simulink model "uz_mpc_6ph"  (R2024b)
settings: Solver=FixedStepDiscrete  StartTime=0.0  StopTime=0.003  RelTol=1e-3
values from neighbouring files (symbols this model uses):
  IB = sqrt(2)*IR    [uz_mpc_6ph_init.m]    (also in uz_mpc_6ph_state_machine_init.m)
  id_ref = 0.0    (= 0)    [uz_mpc_6ph_init.m]    (also in uz_mpc_6ph_state_machine_init.m)
  iq_ref = 15.0    (= 15)    [uz_mpc_6ph_init.m]    (also in uz_mpc_6ph_state_machine_init.m = 3)
  ix_ref = 0.0    (= 0)    [uz_mpc_6ph_init.m]    (also in uz_mpc_6ph_state_machine_init.m)
  iy_ref = 0.0    (= 0)    [uz_mpc_6ph_init.m]    (also in uz_mpc_6ph_state_machine_init.m)
  lambda_d = 1.0    (= 1)    [uz_mpc_6ph_init.m]    (also in uz_mpc_6ph_state_machine_init.m)
  lambda_q = 1.0    (= 1)    [uz_mpc_6ph_init.m]    (also in uz_mpc_6ph_state_machine_init.m)
  lambda_u = 0.0    (= 0)    [uz_mpc_6ph_init.m]    (also in uz_mpc_6ph_state_machine_init.m)
  lambda_x = 1.0    (= 1)    [uz_mpc_6ph_init.m]    (also in uz_mpc_6ph_state_machine_init.m)
  lambda_y = 1.0    (= 1)    [uz_mpc_6ph_init.m]    (also in uz_mpc_6ph_state_machine_init.m)
  Ld_over_LB = Ld/LB    [uz_mpc_6ph_init.m]    (also in uz_mpc_6ph_state_machine_init.m)
  Lq_over_LB = Lq/LB    [uz_mpc_6ph_init.m]    (also in uz_mpc_6ph_state_machine_init.m)
  n_rpm = 2200.0    (= 2200)    [uz_mpc_6ph_init.m]    (also in uz_mpc_6ph_state_machine_init.m = 1200)
  omegaB = nR*2*pi()/60*p    [uz_mpc_6ph_init.m]    (also in uz_mpc_6ph_state_machine_init.m)
  p = 5    [uz_mpc_6ph_init.m]    (also in uz_mpc_6ph_state_machine_init.m)
  psi_pm_over_psiB = psi_pm/psiB    [uz_mpc_6ph_init.m]    (also in uz_mpc_6ph_state_machine_init.m)
  Rs_over_ZB = Rs/ZB    [uz_mpc_6ph_init.m]    (also in uz_mpc_6ph_state_machine_init.m)
  t_ADC = 1/f_ADC    (= 1e-05)    [uz_mpc_6ph_init.m]    (also in uz_mpc_6ph_state_machine_init.m)
  t_clock = 1/f_clock    (= 1e-08)    [uz_mpc_6ph_init.m]    (also in uz_mpc_6ph_state_machine_init.m)
  Ts_times_ZB_over_Ld = Ts*ZB/Ld    [uz_mpc_6ph_init.m]    (also in uz_mpc_6ph_state_machine_init.m)
  Ts_times_ZB_over_Lq = Ts*ZB/Lq    [uz_mpc_6ph_init.m]    (also in uz_mpc_6ph_state_machine_init.m)
  Ts_times_ZB_over_Lx = Ts*ZB/Lx    [uz_mpc_6ph_init.m]    (also in uz_mpc_6ph_state_machine_init.m)
  Ts_times_ZB_over_Ly = Ts*ZB/Ly    [uz_mpc_6ph_init.m]    (also in uz_mpc_6ph_state_machine_init.m)
  v_dc = 565.0    (= 565)    [uz_mpc_6ph_init.m]    (also in uz_mpc_6ph_state_machine_init.m)
  VB = sqrt(2/3)*VR    [uz_mpc_6ph_init.m]    (also in uz_mpc_6ph_state_machine_init.m)
libraries: nesl_utility x32, fl_lib x29, simulink x23, ee_lib x12, hdlsllib x2, spsAlphaBetaZerotodq0Lib x1, batteryecm_lib x1
(part 1 of 4)
settings Model: DataTypeOverride=Off  Creator=micha  LastModifiedBy=hufnagelde
settings SolverCC: AlgebraicLoopSolver=TrustRegion
settings DataIOCC: LimitDataPoints=on  SaveOutput=off  SaveTime=off
settings OptimizationCC: BlockReduction=off  ConditionallyExecuteInputs=off  DefaultParameterBehavior=Inlined  LifeSpan=inf
settings DebuggingCC: AlgebraicLoopMsg=error  SingleTaskRateTransMsg=error  UnconnectedInputMsg=warning  UnconnectedOutputMsg=warning  UnconnectedLineMsg=warning  AllowSymbolicDim=off  StrictBusMsg=ErrorOnBusTreatedAsVector  SFUnexpectedBacktrackingDiag=warning  SFNoUnconditionalDefaultTransitionDiag=warning  SFExecutionAtInitializationDiag=none  ArithmeticOperatorsInVariantConditions=warning
settings HardwareCC: ProdBitPerPointer=32  ProdBitPerSizeT=32  ProdBitPerPtrDiffT=32  ProdLargestAtomicFloat=None  ProdIntDivRoundTo=Undefined  ProdEndianess=Unspecified  ProdWordSize=32  ProdHWDeviceType=ASIC/FPGA->ASIC/FPGA  ProdEqTarget=off
settings ModelReferenceCC: EnableRefExpFcnMdlSchedulingChecks=on
settings SFSimCC: SimUseLocalCustomCode=off  CustomCodeUndefinedFunction=UseInterfaceOnly
settings RTWCC: RTWUseLocalCustomCode=off  GPUComputeCapability=3.5  DLArmComputeVersion=19.05
settings CodeAppCC: StateflowObjectComments=on
settings GRTTargetCC: TargetLangStandard=C89/C90 (ANSI)
settings ConfigComp: CovScope=ReferencedModels  CovMetricSettings=dw  CovSaveCumulativeToWorkspaceVar=on  CovSaveSingleToWorkspaceVar=on  CovExternalEMLEnable=off  CovSFcnEnable=off

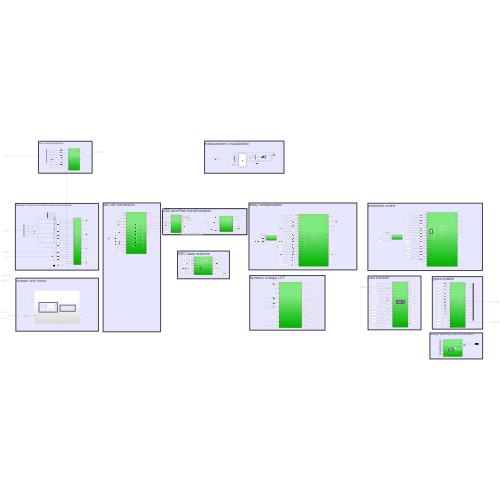
[thumbnail: Simulink's stored preview of the top-level diagram]
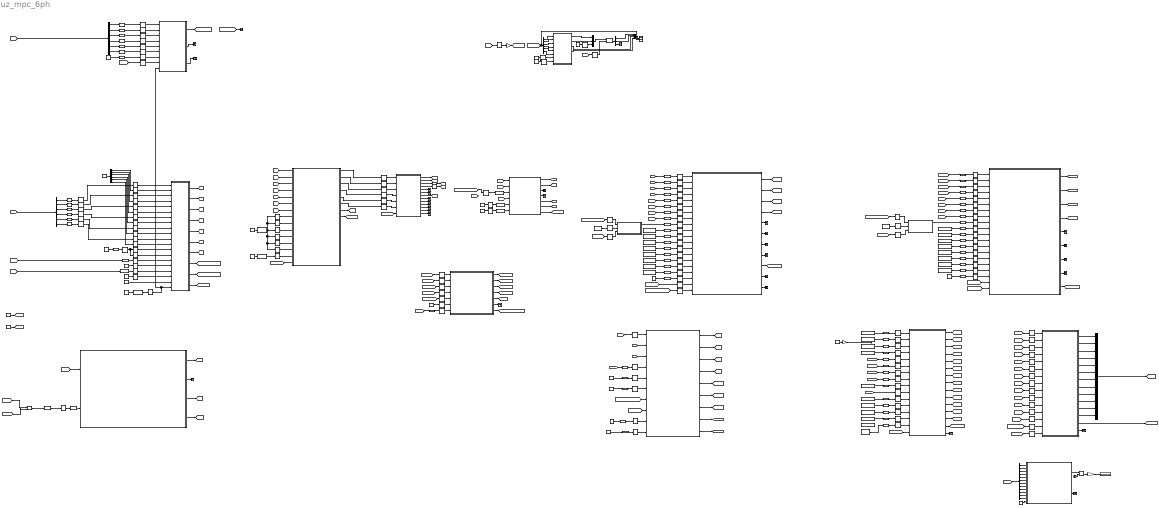
== system uz_mpc_6ph ==
  note: measurement visualization
  note: sfix27_En24 = +-4 p.u.
  note: current limit in A
  note: inverter and motor
  note: debug ip for input of constant measurement values
  note: VSD and Park transformation
  note: MPC state machine
  note: per unit conversion
  note: average switching frequency calculation
  note: gates enable
  note: cost function
  note: prediction model
  note: dynamic voltage LUT
  note: delay compensation
  note: 1=real 0=debug
  note: 5 steps delay for xy currents, since dq transformation of alpha beta currents takes 5 clock steps. This way, the delay of dq is compensated. For implementation not relevant!
  note: 0=AXI 1=PL
  note: 0=AXI 1=PL
  note: over current protection
  6ph_PMSM_30deg_VSD1 : MATLAB Function  TreatAsAtomicUnit=on
  AND : Logic  IconShape=distinctive  AllPortsSameDT=off  OutDataTypeStr=boolean
  Alpha-Beta-Zero to dq1 : spsAlphaBetaZerotodq0Lib/Alpha-Beta-Zero to dq0  Alignment=Aligned with phase A axis
  Clock : Clock
  Constant : Constant  Value=64  OutDataTypeStr=uint32  SampleTime=-1
  Constant1 : Constant  Value=p
  Constant10 : Constant  Value=psi_pm_over_psiB
  Constant11 : Constant  Value=1.2
  Constant12 : Constant  Value=0
  Constant13 : Constant  Value=p
  Constant14 : Constant  Value=psi_pm_over_psiB
  Constant15 : Constant  Value=Rs_over_ZB
  Constant16 : Constant  Value=12
  Constant17 : Constant  Value=Ts_times_ZB_over_Ld
  Constant18 : Constant  Value=Ts_times_ZB_over_Lq
  Constant19 : Constant  Value=Ts_times_ZB_over_Lx
  Constant{2,25,51,62} (4 alike) : Constant
  Constant20 : Constant  Value=Ts_times_ZB_over_Ly
  Constant21 : Constant  Value=Ld_over_LB
  Constant22 : Constant  Value=Lq_over_LB
  Constant23 : Constant  Value=39
  Constant24 : Constant  Value=1/3
  Constant26 : Constant  Value=v_dc
  Constant27 : Constant  Value=iq_ref/IB
  Constant28 : Constant  Value=ix_ref/IB
  Constant29 : Constant  Value=iy_ref/IB
  Constant3 : Constant  Value=Rs_over_ZB
  Constant30 : Constant  Value=0  SampleTime=-1
  Constant31 : Constant  Value=lambda_d
  Constant32 : Constant  Value=lambda_q
  Constant33 : Constant  Value=lambda_x
  Constant34 : Constant  Value=lambda_y
  Constant35 : Constant  Value=lambda_u
  Constant36 : Constant  OutDataTypeStr=boolean  SampleTime=-1
  Constant37 : Constant  OutDataTypeStr=boolean  SampleTime=-1
  Constant4 : Constant  Value=Ts_times_ZB_over_Ld
  Constant42 : Constant  Value=id_ref/IB
  Constant44 : Constant  Value=0  SampleTime=-1
  Constant5 : Constant  Value=Ts_times_ZB_over_Lq
  Constant52 : Constant  Value=0
  Constant53 : Constant  Value=1/omegaB  OutDataTypeStr=fixdt(0,18,18)
  Constant54 : Constant  Value=1/omegaB  OutDataTypeStr=fixdt(0,18,18)
  Constant55 : Constant  Value=0  OutDataTypeStr=fixdt(1,24,11)  SampleTime=-1
  Constant56 : Constant  Value=1/IB
  Constant57 : Constant  Value=1/VB
  Constant58 : Constant  Value=63
  Constant59 : Constant  OutDataTypeStr=boolean  SampleTime=-1
  Constant6 : Constant  Value=Ts_times_ZB_over_Lx
  Constant60 : Constant  Value=[1 2 3 4 5 6]  OutDataTypeStr=fixdt(1,27,15)  SampleTime=-1
  Constant61 : Constant  Value=0  OutDataTypeStr=fixdt(1,27,20)  SampleTime=-1
  Constant63 : Constant  Value=0.15
  Constant7 : Constant  Value=Ts_times_ZB_over_Ly
  Constant8 : Constant  Value=Ld_over_LB
  Constant9 : Constant  Value=Lq_over_LB
  Data Type Conversion{,3,55..58} (6 alike) : DataTypeConversion  OutDataTypeStr=fixdt_type_xy_currents  SaturateOnIntegerOverflow=off  RndMeth=Floor
  Data Type Conversion1 : DataTypeConversion  OutDataTypeStr=boolean  SaturateOnIntegerOverflow=off  RndMeth=Floor
  Data Type Conversion{2,6,10..11,13,65..66} (7 alike) : DataTypeConversion  OutDataTypeStr=fixdt_type_polepairs  SaturateOnIntegerOverflow=off  RndMeth=Floor
  Data Type Conversion{12,14..28} (16 alike) : DataTypeConversion  OutDataTypeStr=fixdt_type_constants  SaturateOnIntegerOverflow=off  RndMeth=Floor
  Data Type Conversion29 : DataTypeConversion  OutDataTypeStr=fixdt_type_speed  SaturateOnIntegerOverflow=off  RndMeth=Floor
  Data Type Conversion30 : DataTypeConversion  OutDataTypeStr=fixdt_type_speed  SaturateOnIntegerOverflow=off  RndMeth=Floor
  Data Type Conversion{4..5,31,43..45,50..53} (10 alike) : DataTypeConversion  OutDataTypeStr=fixdt_type_dq_currents  SaturateOnIntegerOverflow=off  RndMeth=Floor
  Data Type Conversion32 : DataTypeConversion  OutDataTypeStr=fixdt(0,18,18)  SaturateOnIntegerOverflow=off  RndMeth=Floor
  Data Type Conversion33 : DataTypeConversion  OutDataTypeStr=fixdt(0,18,18)  SaturateOnIntegerOverflow=off  RndMeth=Floor
  Data Type Conversion{34..36,38,40,67..68,71..77} (14 alike) : DataTypeConversion  OutDataTypeStr=fixdt(1,27,15)  SaturateOnIntegerOverflow=off  RndMeth=Floor
  Data Type Conversion37 : DataTypeConversion  OutDataTypeStr=fixdt(1,27,20)  SaturateOnIntegerOverflow=off  RndMeth=Floor
  Data Type Conversion39 : DataTypeConversion  OutDataTypeStr=fixdt(1,18,14)  SaturateOnIntegerOverflow=off  RndMeth=Floor
  Data Type Conversion{7..8,41..42,46..49} (8 alike) : DataTypeConversion  OutDataTypeStr=fixdt_type_dqxy_voltages  SaturateOnIntegerOverflow=off  RndMeth=Floor
  Data Type Conversion54 : DataTypeConversion  OutDataTypeStr=fixdt_type_max_current  SaturateOnIntegerOverflow=off  RndMeth=Floor
  Data Type Conversion59 : DataTypeConversion  OutDataTypeStr=fixdt(1,18,14)  SaturateOnIntegerOverflow=off  RndMeth=Floor
  Data Type Conversion{60..64} (5 alike) : DataTypeConversion  OutDataTypeStr=fixdt_type_lambda  SaturateOnIntegerOverflow=off  RndMeth=Floor
  Data Type Conversion69 : DataTypeConversion  OutDataTypeStr=fixdt(1,24,11)  SaturateOnIntegerOverflow=off  RndMeth=Floor
  Data Type Conversion70 : DataTypeConversion  OutDataTypeStr=fixdt(1,18,15)  SaturateOnIntegerOverflow=off  RndMeth=Floor
  Data Type Conversion78 : DataTypeConversion  OutDataTypeStr=double  SaturateOnIntegerOverflow=off  RndMeth=Floor
  Data Type Conversion79 : DataTypeConversion  OutDataTypeStr=boolean  SaturateOnIntegerOverflow=off  RndMeth=Floor
  Data Type Conversion9 : DataTypeConversion  OutDataTypeStr=fixdt(1,27,20)  SaturateOnIntegerOverflow=off  RndMeth=Floor
  Delay3 : Delay  DelayLength=5
  Delay4 : Delay  DelayLength=5
  Demux{,1,5..6} (4 alike) : Demux  Outputs=6
  Demux2 : Demux  Outputs=12
  Demux4 : Demux  Outputs=3
  Display : Display
  Divide : Product  Inputs=*/
  Gain : Gain  Gain=1/IB
  Gain1 : Gain  Gain=1/IB
  Gain19 : Gain  Gain=1/(12*2)
  Mux : Mux
  Mux2 : Mux  Inputs=12
  Mux5 : Mux  Inputs=3
  Pulse Generator2 : DiscretePulseGenerator  PulseType=Time based  Period=t_ADC  PulseWidth=5
  Rate Transition{,5,8,131..132} (5 alike) : RateTransition  OutPortSampleTime=t_ADC
  Rate Transition{1..4,6..7,9..10,12..54,56..67,69..74,77..128,130,133..141} (131 alike) : RateTransition  OutPortSampleTime=t_clock
  Rate Transition{11,55,68,75..76,129} (6 alike) : RateTransition  InitialCondition=1  OutPortSampleTime=t_clock
  Scope : Scope  NumInputPorts=2
  Terminator{,1..28} (29 alike) : Terminator
  Transport Delay : TransportDelay  DelayTime=0.0015  InitialOutput=1
  cost_opt : Subsystem  TreatAsAtomicUnit=on
  counter_f_sw_6ph : Subsystem
  ctrl_state_machine : Subsystem  TreatAsAtomicUnit=on
  delay_comp : Subsystem  TreatAsAtomicUnit=on
  inverter_machine : Subsystem
  mpc_enable : Subsystem  TreatAsAtomicUnit=on
  prediction : Subsystem  TreatAsAtomicUnit=on
  pu_omega_m : Subsystem  TreatAsAtomicUnit=on
  pu_omega_m1 : Subsystem
  pu_voltages_vsd : Subsystem  TreatAsAtomicUnit=on
  uz_current_limit : Subsystem  TreatAsAtomicUnit=on
  uz_debug_switch_measurements : Subsystem  TreatAsAtomicUnit=on
  uz_park_transformation : Subsystem  TreatAsAtomicUnit=on
  uz_pu_conversion : Subsystem  TreatAsAtomicUnit=on
  uz_vsd_6ph_30deg : Subsystem  TreatAsAtomicUnit=on
  wires:
  [optimization_done] -> Rate Transition4/1
  [prediction_done] -> Rate Transition3/1
  [delay_comp_done] -> Rate Transition2/1
  [voltages_done] -> Rate Transition1/1
  Rate Transition58/1 -> ctrl_state_machine/1(trigger_start_state_machine)  "park_done"
  Rate Transition1/1 -> ctrl_state_machine/2(trigger_voltages_done)  "volts_done"
  Rate Transition2/1 -> ctrl_state_machine/3(trigger_delay_comp_done)  "delay_done"
  Rate Transition3/1 -> ctrl_state_machine/4(trigger_prediction_done)  "pred_done"
  Rate Transition4/1 -> ctrl_state_machine/5(trigger_optimization_done)  "opt_done"
  Rate Transition9/1 -> ctrl_state_machine/6(AXI_no_of_iterations)  "opt_done"
  Constant/1 -> Rate Transition9/1
  uz_park_transformation/7(park_done) -> [trigger_park_done]  "calc_done"
  Rate Transition36/1 -> uz_vsd_6ph_30deg/5(b2)
  Rate Transition38/1 -> Data Type Conversion9/1
  Data Type Conversion39/1 -> uz_park_transformation/5(factor_angle_el_AXI)
  uz_park_transformation/3(y1_AXI) -> Terminator8/1
  uz_vsd_6ph_30deg/8(alpha_AXI) -> Terminator2/1
  Data Type Conversion9/1 -> uz_park_transformation/3(angle_el)
  uz_park_transformation/2(y2) -> [iq_pu]  "iq_pu"
  Data Type Conversion59/1 -> uz_park_transformation/6(offset_angle_el_AXI)
  uz_vsd_6ph_30deg/3(x1) -> Delay3/1
  Demux/4 -> Data Type Conversion38/1
  Rate Transition61/1 -> Data Type Conversion59/1
  Rate Transition40/1 -> Data Type Conversion39/1
  uz_vsd_6ph_30deg/4(y1) -> Delay4/1
  Constant12/1 -> Rate Transition61/1
  uz_vsd_6ph_30deg/5(z1) -> Terminator/1
  uz_vsd_6ph_30deg/6(z2) -> Terminator1/1
  uz_vsd_6ph_30deg/13(z2_AXI) -> Terminator7/1
  Demux/2 -> Data Type Conversion35/1
  Rate Transition33/1 -> uz_vsd_6ph_30deg/3(c1)
  uz_park_transformation/1(y1) -> [id_pu]  "id_pu"
  uz_vsd_6ph_30deg/10(x_AXI) -> Terminator4/1
  inverter_machine/4(omega_m) -> [omega_m]
  inverter_machine/3(theta_el) -> [theta_el]
  inverter_machine/2(i_dc) -> Terminator25/1
  uz_vsd_6ph_30deg/9(beta_AXI) -> Terminator3/1
  uz_park_transformation/5(sin) -> [sin]
  inverter_machine/1(i_ph) -> [i_ph]
  uz_vsd_6ph_30deg/12(z1_AXI) -> Terminator6/1
  [i_ph] -> Demux/1
  Rate Transition35/1 -> uz_vsd_6ph_30deg/1(a1)
  Constant25/1 -> Rate Transition40/1
  Demux/6 -> Data Type Conversion67/1
  Demux/5 -> Data Type Conversion40/1
  Demux/3 -> Data Type Conversion36/1
  Rate Transition32/1 -> uz_vsd_6ph_30deg/2(b1)
  Demux/1 -> Data Type Conversion34/1
  uz_pu_conversion/8(pu_conv_done) -> [pu_conv_valid]
  Data Type Conversion1/1 -> Rate Transition10/1
  uz_vsd_6ph_30deg/11(y_AXI) -> Terminator5/1
  Rate Transition34/1 -> uz_vsd_6ph_30deg/4(a2)
  Pulse Generator2/1 -> Data Type Conversion1/1
  uz_park_transformation/6(cos) -> [cos]
  [theta_el_from_debug_switch] -> Rate Transition38/1
  uz_park_transformation/4(y2_AXI) -> Terminator9/1
  Constant13/1 -> Data Type Conversion11/1
  Constant14/1 -> Data Type Conversion27/1
  Data Type Conversion16/1 -> Rate Transition14/1
  Data Type Conversion12/1 -> Rate Transition13/1
  Data Type Conversion65/1 -> Rate Transition55/1
  Rate Transition15/1 -> delay_comp/18(polepairs_AXI)
  pu_voltages_vsd/9(voltages_done) -> [voltages_done]  "calc_done"
  pu_voltages_vsd/1(pu_vd) -> [vd_pu]
  [v_dc_pu] -> Rate Transition46/1
  Constant22/1 -> Data Type Conversion19/1
  Rate Transition74/1 -> delay_comp/6(vq_pu)
  Rate Transition47/1 -> delay_comp/7(vx_pu)
  Data Type Conversion41/1 -> Rate Transition47/1
  Rate Transition51/1 -> prediction/7(vx_pu)
  Data Type Conversion14/1 -> Rate Transition20/1
  Rate Transition19/1 -> prediction/17(psi_pm_over_psiB_AXI)
  Constant15/1 -> Data Type Conversion12/1
  Constant21/1 -> Data Type Conversion18/1
  Constant18/1 -> Data Type Conversion15/1
  pu_omega_m1/1(out1) -> Data Type Conversion30/1
  Data Type Conversion21/1 -> Rate Transition39/1
  Constant8/1 -> Data Type Conversion25/1
  Rate Transition75/1 -> pu_voltages_vsd/4(index)
  [vq_pu] -> Data Type Conversion8/1
  delay_comp/9(delay_comp_done) -> [delay_comp_done]
  Data Type Conversion18/1 -> Rate Transition17/1
  pu_voltages_vsd/2(pu_vq) -> [vq_pu]
  Data Type Conversion45/1 -> Rate Transition50/1
  Rate Transition24/1 -> prediction/4(iy_delay_pu)
  Rate Transition26/1 -> delay_comp/13(Ts_times_ZB_over_Lx_AXI)
  Constant2/1 -> Data Type Conversion2/1
  [cos] -> pu_voltages_vsd/3(cos_angle)
  Rate Transition46/1 -> pu_voltages_vsd/1(v_DC_pu)
  Constant30/1 -> counter_f_sw_6ph/13(bResetAXI)
  Data Type Conversion31/1 -> Rate Transition49/1
  [iq_delay_pu] -> Data Type Conversion45/1
  Data Type Conversion15/1 -> Rate Transition21/1
  counter_f_sw_6ph/1(switchNumb_AXI) -> Divide/1
  Rate Transition48/1 -> delay_comp/8(vy_pu)
  Rate Transition21/1 -> prediction/12(Ts_times_ZB_over_Lq_AXI)
  Constant17/1 -> Data Type Conversion14/1
  pu_voltages_vsd/5(pu_vd_AXI) -> [vd_pu_AXI]
  Data Type Conversion47/1 -> Rate Transition52/1
  Rate Transition50/1 -> prediction/2(iq_delay_pu)
  cost_opt/15(costs) -> Terminator10/1
  Rate Transition67/1 -> delay_comp/5(vd_pu)
  Demux2/11 -> counter_f_sw_6ph/11(ss_in_10)
  [opt_gates] -> Demux2/1
  Data Type Conversion30/1 -> Rate Transition23/1
  Demux2/2 -> counter_f_sw_6ph/2(ss_in_1)
  Rate Transition44/1 -> delay_comp/3(ix_pu)
  Constant9/1 -> Data Type Conversion26/1
  Clock/1 -> Divide/2
  Data Type Conversion42/1 -> Rate Transition48/1
  Demux2/3 -> counter_f_sw_6ph/3(ss_in_2)
  Demux2/10 -> counter_f_sw_6ph/10(ss_in_9)
  Data Type Conversion58/1 -> Rate Transition66/1
  Data Type Conversion4/1 -> Rate Transition41/1
  [index] -> Data Type Conversion6/1
  Demux2/1 -> counter_f_sw_6ph/1(ss_in_0)
  Rate Transition18/1 -> prediction/16(Lq_over_LB_AXI)
  Rate Transition68/1 -> cost_opt/10(index)
  Rate Transition52/1 -> prediction/8(vy_pu)
  pu_voltages_vsd/3(pu_vx) -> [vx_pu]
  Data Type Conversion57/1 -> Rate Transition65/1
  Rate Transition11/1 -> pu_voltages_vsd/5(index_select_AXI)
  Demux2/6 -> counter_f_sw_6ph/6(ss_in_5)
  Constant20/1 -> Data Type Conversion17/1
  Gain19/1 -> Display/1
  Data Type Conversion28/1 -> Rate Transition31/1
  Demux2/12 -> counter_f_sw_6ph/12(ss_in_11)
  Rate Transition69/1 -> cost_opt/11(lambda_d_AXI)
  Rate Transition54/1 -> prediction/6(vq_pu)
  [sin] -> pu_voltages_vsd/2(sin_angle)
  Demux2/7 -> counter_f_sw_6ph/7(ss_in_6)
  prediction/4(iy_pred_pu) -> [iy_pred_pu]
  Demux2/8 -> counter_f_sw_6ph/8(ss_in_7)
  pu_voltages_vsd/7(pu_vx_AXI) -> [vx_pu_AXI]
  Rate Transition70/1 -> cost_opt/12(lambda_q_AXI)
  pu_voltages_vsd/6(pu_vq_AXI) -> [vq_pu_AXI]
  [index] -> Rate Transition68/1
  Data Type Conversion27/1 -> Rate Transition19/1
  pu_voltages_vsd/8(pu_vy_AXI) -> [vy_pu_AXI]
  [vd_pu] -> Data Type Conversion7/1
  Data Type Conversion43/1 -> Rate Transition24/1
  Constant32/1 -> Data Type Conversion61/1
  Constant11/1 -> Data Type Conversion54/1
  Data Type Conversion19/1 -> Rate Transition18/1
  Data Type Conversion10/1 -> Rate Transition76/1
  Constant19/1 -> Data Type Conversion16/1
  Data Type Conversion48/1 -> Rate Transition53/1
  Rate Transition12/1 -> prediction/18(polepairs_AXI)
  Rate Transition20/1 -> prediction/11(Ts_times_ZB_over_Ld_AXI)
  Rate Transition29/1 -> delay_comp/15(Ld_over_LB_AXI)
  Rate Transition17/1 -> prediction/15(Ld_over_LB_AXI)
  pu_voltages_vsd/4(pu_vy) -> [vy_pu]
  Data Type Conversion13/1 -> Rate Transition15/1
  [opt_index] -> Data Type Conversion10/1
  Rate Transition22/1 -> delay_comp/4(iy_pu)
  Rate Transition43/1 -> delay_comp/9(omega_m_pu)
  Data Type Conversion11/1 -> Rate Transition12/1
  Constant10/1 -> Data Type Conversion28/1
  Data Type Conversion51/1 -> Rate Transition56/1
  [iy_pu] -> Data Type Conversion3/1
  [vd_pu] -> Data Type Conversion48/1
  Data Type Conversion17/1 -> Rate Transition16/1
  Data Type Conversion46/1 -> Rate Transition51/1
  Data Type Conversion3/1 -> Rate Transition22/1
  Constant1/1 -> Data Type Conversion13/1
  prediction/9(prediction_done) -> [prediction_done]
  Constant33/1 -> Data Type Conversion62/1
  Rate Transition53/1 -> prediction/5(vd_pu)
  cost_opt/1(opt_index) -> [opt_index]  "result"
  Rate Transition13/1 -> prediction/10(Rs_over_ZB_AXI)
  [iq_pu] -> Data Type Conversion5/1
  Constant34/1 -> Data Type Conversion63/1
  Data Type Conversion20/1 -> Rate Transition25/1
  Rate Transition60/1 -> cost_opt/6(iq_pred_pu)
  cost_opt/14(optimization_done) -> [optimization_done]  "optimization done"
  Data Type Conversion56/1 -> Rate Transition64/1
  Constant44/1 -> Data Type Conversion64/1
  Constant4/1 -> Data Type Conversion21/1
  Rate Transition73/1 -> cost_opt/15(lambda_u_AXI)
  Data Type Conversion64/1 -> Rate Transition73/1
  Demux2/4 -> counter_f_sw_6ph/4(ss_in_3)
  Data Type Conversion61/1 -> Rate Transition70/1
  Data Type Conversion22/1 -> Rate Transition42/1
  Rate Transition76/1 -> ctrl_state_machine/7(last_opt_index)
  Data Type Conversion60/1 -> Rate Transition69/1
  Constant42/1 -> Data Type Conversion57/1
  Rate Transition71/1 -> cost_opt/13(lambda_x_AXI)
  Rate Transition72/1 -> cost_opt/14(lambda_y_AXI)
  Rate Transition63/1 -> cost_opt/3(ix_ref_pu_AXI)
  Constant5/1 -> Data Type Conversion22/1
  Rate Transition64/1 -> cost_opt/4(iy_ref_pu_AXI)
  Rate Transition65/1 -> cost_opt/1(id_ref_pu_AXI)
  Rate Transition16/1 -> prediction/14(Ts_times_ZB_over_Ly_AXI)
  [vy_pu] -> Data Type Conversion42/1
  Divide/1 -> Gain19/1
  [vx_pu] -> Data Type Conversion41/1
  Rate Transition57/1 -> cost_opt/5(id_pred_pu)
  Rate Transition23/1 -> prediction/9(omega_m_pu)
  Gain1/1 -> ?
  Data Type Conversion6/1 -> Rate Transition75/1
  [iq_pred_pu] -> Data Type Conversion53/1
  Rate Transition28/1 -> prediction/1(id_delay_pu)
  Rate Transition55/1 -> pu_voltages_vsd/6(index_AXI)
  Data Type Conversion63/1 -> Rate Transition72/1
  Constant6/1 -> Data Type Conversion23/1
  Rate Transition59/1 -> cost_opt/7(ix_pred_pu)
  Data Type Conversion55/1 -> Rate Transition63/1
  Data Type Conversion44/1 -> Rate Transition28/1
  [ix_pred_pu] -> Data Type Conversion50/1
  [id_pred_pu] -> Data Type Conversion52/1
  Rate Transition31/1 -> delay_comp/17(psi_pm_over_psiB_AXI)
  Data Type Conversion52/1 -> Rate Transition57/1
  Data Type Conversion49/1 -> Rate Transition54/1
  Data Type Conversion8/1 -> Rate Transition74/1
  [id_delay_pu] -> Data Type Conversion44/1
  [id_pu] -> Data Type Conversion4/1
  Data Type Conversion62/1 -> Rate Transition71/1
  [iy_delay_pu] -> Data Type Conversion43/1
  Rate Transition66/1 -> cost_opt/2(iq_ref_pu_AXI)
  [ix_delay_pu] -> Data Type Conversion31/1
  Data Type Conversion53/1 -> Rate Transition60/1
  counter_f_sw_6ph/2(switchNumb) -> Terminator24/1
  [ix_pu] -> Data Type Conversion/1
  Data Type Conversion54/1 -> Rate Transition62/1
  prediction/3(ix_pred_pu) -> [ix_pred_pu]
  Data Type Conversion24/1 -> Rate Transition27/1
  [vx_pu] -> Data Type Conversion46/1
  [iy_pred_pu] -> Data Type Conversion51/1
  [vq_pu] -> Data Type Conversion49/1
  Data Type Conversion2/1 -> Rate Transition11/1
  prediction/1(id_pred_pu) -> [id_pred_pu]
  Constant28/1 -> Data Type Conversion55/1
  Data Type Conversion/1 -> Rate Transition44/1
  Rate Transition25/1 -> delay_comp/10(Rs_over_ZB_AXI)
  Demux2/5 -> counter_f_sw_6ph/5(ss_in_4)
  [vy_pu] -> Data Type Conversion47/1
  Data Type Conversion5/1 -> Rate Transition45/1
  Data Type Conversion23/1 -> Rate Transition26/1
  Constant3/1 -> Data Type Conversion20/1
  Data Type Conversion26/1 -> Rate Transition30/1
  Rate Transition27/1 -> delay_comp/14(Ts_times_ZB_over_Ly_AXI)
  Rate Transition42/1 -> delay_comp/12(Ts_times_ZB_over_Lq_AXI)
  Rate Transition14/1 -> prediction/13(Ts_times_ZB_over_Lx_AXI)
  Constant31/1 -> Data Type Conversion60/1
  Rate Transition30/1 -> delay_comp/16(Lq_over_LB_AXI)
  Data Type Conversion25/1 -> Rate Transition29/1
  Rate Transition56/1 -> cost_opt/8(iy_pred_pu)
  Demux2/9 -> counter_f_sw_6ph/9(ss_in_8)
  Data Type Conversion50/1 -> Rate Transition59/1
  Data Type Conversion7/1 -> Rate Transition67/1
  Constant7/1 -> Data Type Conversion24/1
  pu_omega_m/1(out1) -> Data Type Conversion29/1
  Rate Transition45/1 -> delay_comp/2(iq_pu)
  Rate Transition49/1 -> prediction/3(ix_delay_pu)
  Data Type Conversion29/1 -> Rate Transition43/1
  Rate Transition62/1 -> cost_opt/9(max_current_pu_AXI)
  Rate Transition39/1 -> delay_comp/11(Ts_times_ZB_over_Ld_AXI)
  Constant29/1 -> Data Type Conversion56/1
  [trigger_park_done] -> Rate Transition58/1
  [delay_comp_done] -> prediction/20(trigger_delay_comp_done)
  [trigger_park_done_statemachine] -> pu_voltages_vsd/7(trigger_park_done)
  ctrl_state_machine/5(index) -> [index]
  Rate Transition37/1 -> uz_vsd_6ph_30deg/6(c2)
  Rate Transition41/1 -> delay_comp/1(id_pu)  "id_measured"
  [opt_gates] -> inverter_machine/1(In1)
  delay_comp/1(id_delay_pu) -> [id_delay_pu]  "id_delay"
  delay_comp/2(iq_delay_pu) -> [iq_delay_pu]
  delay_comp/4(iy_delay_pu) -> [iy_delay_pu]
  delay_comp/3(ix_delay_pu) -> [ix_delay_pu]
  ctrl_state_machine/7(trigger_park_done_statemachine) -> [trigger_park_done_statemachine]
  [trigger_park_done_statemachine] -> Rate Transition6/1
  Rate Transition6/1 -> delay_comp/20(trigger_park_done)
  Rate Transition7/1 -> delay_comp/19(trigger_delay_comp)
  Delay3/1 -> [ix_pu]
  Delay4/1 -> [iy_pu]
  Demux5/4 -> 6ph_PMSM_30deg_VSD1/4(u4)
  Demux5/5 -> 6ph_PMSM_30deg_VSD1/5(u5)
  Demux5/2 -> 6ph_PMSM_30deg_VSD1/2(u2)
  Demux5/3 -> 6ph_PMSM_30deg_VSD1/3(u3)
  Constant51/1 -> Rate Transition8/1
  [pu_phase_currents] -> Scope/2, Demux5/1
  Constant24/1 -> Rate Transition5/1
  Demux5/1 -> 6ph_PMSM_30deg_VSD1/1(u1)
  Demux5/6 -> 6ph_PMSM_30deg_VSD1/6(u6)
  [i_ph] -> Rate Transition/1
  Gain/1 -> [pu_phase_currents]
  Constant52/1 -> Rate Transition131/1
  [theta_el] -> Rate Transition132/1
  6ph_PMSM_30deg_VSD1/1(y1) -> Mux5/1  "alpha"
  Mux5/1 -> Alpha-Beta-Zero to dq1/1
  Alpha-Beta-Zero to dq1/1 -> Demux4/1
  6ph_PMSM_30deg_VSD1/2(y2) -> Mux5/2  "beta"
  Demux4/3 -> Terminator11/1
  [omega_m_from_debug_switch] -> Rate Transition79/1
  [pu_conv_valid] -> Rate Transition77/1
  Constant53/1 -> Rate Transition78/1
  Rate Transition77/1 -> pu_omega_m/3(adc_valid_trigger)
  Rate Transition78/1 -> pu_omega_m/2(AXI_pu_conv_in)
  Rate Transition79/1 -> pu_omega_m/1(in1)
  Rate Transition80/1 -> pu_omega_m1/3(adc_valid_trigger)
  Rate Transition82/1 -> pu_omega_m1/1(in1)
  [pu_conv_valid] -> Rate Transition80/1
  Constant54/1 -> Rate Transition81/1
  Rate Transition81/1 -> pu_omega_m1/2(AXI_pu_conv_in)
  [omega_m_from_debug_switch] -> Rate Transition82/1
  mpc_enable/10(out_G9) -> Mux2/10
  Mux2/1 -> [opt_gates]
  mpc_enable/1(out_G0) -> Mux2/1
  mpc_enable/2(out_G1) -> Mux2/2
  mpc_enable/5(out_G4) -> Mux2/5
  mpc_enable/3(out_G2) -> Mux2/3
  mpc_enable/6(out_G5) -> Mux2/6
  mpc_enable/12(out_G11) -> Mux2/12
  mpc_enable/7(out_G6) -> Mux2/7
  mpc_enable/11(out_G10) -> Mux2/11
  mpc_enable/9(out_G8) -> Mux2/9
  mpc_enable/4(out_G3) -> Mux2/4
  mpc_enable/8(out_G7) -> Mux2/8
  [pu_conv_valid] -> Rate Transition86/1
  [MPC_enb] -> Rate Transition85/1
  Rate Transition83/1 -> mpc_enable/11(G10)
  Rate Transition84/1 -> mpc_enable/12(G11)
  Rate Transition85/1 -> mpc_enable/13(AXI_mpc_enb)
  Rate Transition86/1 -> mpc_enable/15(adc_valid_trigger)
  Rate Transition87/1 -> mpc_enable/9(G8)
  Rate Transition88/1 -> mpc_enable/10(G9)
  Rate Transition89/1 -> mpc_enable/7(G6)
  Rate Transition90/1 -> mpc_enable/8(G7)
  Rate Transition91/1 -> mpc_enable/5(G4)
  Rate Transition92/1 -> mpc_enable/6(G5)
  Rate Transition94/1 -> mpc_enable/4(G3)
  Rate Transition93/1 -> mpc_enable/3(G2)
  Rate Transition95/1 -> mpc_enable/1(G0)
  Rate Transition96/1 -> mpc_enable/2(G1)
  Constant26/1 -> Data Type Conversion68/1
  Rate Transition106/1 -> uz_pu_conversion/8(AXI_pu_conv_in0)
  Rate Transition105/1 -> uz_pu_conversion/9(AXI_pu_conv_in1)
  Rate Transition104/1 -> uz_pu_conversion/10(AXI_pu_conv_in2)
  Rate Transition110/1 -> uz_pu_conversion/11(AXI_pu_conv_in3)
  Rate Transition109/1 -> uz_pu_conversion/12(AXI_pu_conv_in4)
  Rate Transition108/1 -> uz_pu_conversion/13(AXI_pu_conv_in5)
  Rate Transition107/1 -> uz_pu_conversion/14(AXI_pu_conv_in6)
  Constant56/1 -> Data Type Conversion33/1
  Constant57/1 -> Data Type Conversion32/1
  Data Type Conversion32/1 -> Rate Transition107/1
  Data Type Conversion33/1 -> Rate Transition106/1, Rate Transition105/1, Rate Transition104/1, Rate Transition110/1, Rate Transition109/1, Rate Transition108/1
  Data Type Conversion34/1 -> Rate Transition102/1
  Data Type Conversion35/1 -> Rate Transition101/1
  Data Type Conversion36/1 -> Rate Transition100/1
  Data Type Conversion38/1 -> Rate Transition99/1
  Data Type Conversion40/1 -> Rate Transition98/1
  Data Type Conversion67/1 -> Rate Transition97/1
  Data Type Conversion68/1 -> Rate Transition103/1
  uz_pu_conversion/7(out6) -> [v_dc_pu]
  Constant58/1 -> Data Type Conversion65/1
  uz_pu_conversion/1(out0) -> Rate Transition35/1
  uz_pu_conversion/2(out1) -> Rate Transition32/1
  uz_pu_conversion/3(out2) -> Rate Transition33/1
  uz_pu_conversion/4(out3) -> Rate Transition34/1
  uz_pu_conversion/5(out4) -> Rate Transition36/1
  uz_pu_conversion/6(out5) -> Rate Transition37/1
  Rate Transition102/1 -> Rate Transition112/1
  Rate Transition101/1 -> Rate Transition115/1
  Rate Transition100/1 -> Rate Transition114/1
  Rate Transition99/1 -> Rate Transition117/1
  Rate Transition98/1 -> Rate Transition119/1
  Rate Transition97/1 -> Rate Transition121/1
  Rate Transition103/1 -> Rate Transition124/1, Rate Transition123/1
  Rate Transition10/1 -> uz_debug_switch_measurements/20(adc_valid_trigger), uz_current_limit/9(trigger)
  Constant59/1 -> uz_debug_switch_measurements/19(real_or_debug_AXI)
  Rate Transition111/1 -> uz_debug_switch_measurements/2(in0_AXI)
  Rate Transition112/1 -> uz_debug_switch_measurements/1(in0)
  Rate Transition113/1 -> uz_debug_switch_measurements/4(in0_AXI1)
  Rate Transition114/1 -> uz_debug_switch_measurements/5(in2)
  Rate Transition115/1 -> uz_debug_switch_measurements/3(in1)
  Rate Transition116/1 -> uz_debug_switch_measurements/6(in0_AXI2)
  Rate Transition117/1 -> uz_debug_switch_measurements/7(in3)
  Rate Transition118/1 -> uz_debug_switch_measurements/8(in0_AXI3)
  Rate Transition119/1 -> uz_debug_switch_measurements/9(in4)
  Rate Transition120/1 -> uz_debug_switch_measurements/10(in0_AXI4)
  Rate Transition121/1 -> uz_debug_switch_measurements/11(in5)
  Rate Transition122/1 -> uz_debug_switch_measurements/12(in0_AXI5)
  Rate Transition123/1 -> uz_debug_switch_measurements/13(in6)
  Rate Transition124/1 -> uz_debug_switch_measurements/14(in0_AXI6)
  Rate Transition125/1 -> uz_debug_switch_measurements/15(in7)
  Rate Transition126/1 -> uz_debug_switch_measurements/16(in0_AXI7)
  [omega_m] -> Data Type Conversion69/1
  uz_debug_switch_measurements/8(out7) -> [omega_m_from_debug_switch]
  Data Type Conversion69/1 -> Rate Transition125/1
  Constant55/1 -> Rate Transition126/1
  [theta_el] -> Data Type Conversion37/1
  Data Type Conversion37/1 -> Rate Transition127/1
  Rate Transition127/1 -> uz_debug_switch_measurements/17(in8)
  Constant61/1 -> Rate Transition128/1
  Rate Transition128/1 -> uz_debug_switch_measurements/18(in0_AXI8)
  uz_debug_switch_measurements/9(out8) -> [theta_el_from_debug_switch]
  Constant60/1 -> Demux6/1
  Demux6/6 -> Rate Transition122/1
  Demux6/5 -> Rate Transition120/1
  Demux6/4 -> Rate Transition118/1
  Demux6/3 -> Rate Transition116/1
  Demux6/2 -> Rate Transition113/1
  Demux6/1 -> Rate Transition111/1
  Data Type Conversion66/1 -> Rate Transition129/1
  Constant62/1 -> Data Type Conversion66/1
  Rate Transition129/1 -> pu_voltages_vsd/10(v_dc_select_AXI)
  Rate Transition130/1 -> pu_voltages_vsd/9(v_DC_pu_AXI)
  Data Type Conversion70/1 -> Rate Transition130/1
  Constant63/1 -> Data Type Conversion70/1
  ctrl_state_machine/1(trigger_voltages) -> [trigger_voltages]
  [trigger_voltages] -> pu_voltages_vsd/8(trigger_voltages)
  uz_vsd_6ph_30deg/2(beta) -> [beta]
  uz_vsd_6ph_30deg/1(alpha) -> [alpha]
  [alpha] -> uz_park_transformation/1(u1)
  [beta] -> uz_park_transformation/2(u2)
  [vsd_done] -> uz_park_transformation/4(trigger)
  uz_vsd_6ph_30deg/7(vsd_done) -> [vsd_done]
  [trigger_delay_comp] -> Rate Transition7/1
  ctrl_state_machine/2(trigger_delay_comp) -> [trigger_delay_comp]
  [trigger_prediciton] -> prediction/19(trigger_prediction)
  ctrl_state_machine/3(trigger_prediction) -> [trigger_prediciton]
  [trigger_optimization] -> cost_opt/16(trigger_optimization)
  ctrl_state_machine/4(trigger_optimization) -> [trigger_optimization]
  ctrl_state_machine/6(trigger_state_machine_finished) -> Terminator12/1
  delay_comp/5(id_delay_pu_AXI) -> Terminator13/1
  delay_comp/6(iq_delay_pu_AXI) -> Terminator14/1
  delay_comp/7(ix_delay_pu_AXI) -> Terminator15/1
  delay_comp/8(iy_delay_pu_AXI) -> Terminator16/1
  delay_comp/11(Ts_times_ZB_over_Ld) -> Terminator18/1
  delay_comp/10(Rs_over_ZB) -> Terminator17/1
  prediction/5(id_pred_pu_AXI) -> Terminator19/1
  prediction/6(iq_pred_pu_AXI) -> Terminator20/1
  prediction/7(ix_pred_pu_AXI) -> Terminator21/1
  prediction/8(iy_pred_pu_AXI) -> Terminator22/1
  cost_opt/2(G0) -> [G0]
  [G0] -> Rate Transition95/1
  cost_opt/13(G11) -> [G11]
  cost_opt/12(G10) -> [G10]
  cost_opt/11(G9) -> [G9]
  cost_opt/10(G8) -> [G8]
  cost_opt/9(G7) -> [G7]
  cost_opt/8(G6) -> [G6]
  cost_opt/7(G5) -> [G5]
  cost_opt/6(G4) -> [G4]
  cost_opt/5(G3) -> [G3]
  cost_opt/4(G2) -> [G2]
  cost_opt/3(G1) -> [G1]
  [G8] -> Rate Transition87/1
  [G9] -> Rate Transition88/1
  [G10] -> Rate Transition83/1
  [G11] -> Rate Transition84/1
  [G7] -> Rate Transition90/1
  [G6] -> Rate Transition89/1
  [G5] -> Rate Transition92/1
  [G4] -> Rate Transition91/1
  [G3] -> Rate Transition94/1
  [G2] -> Rate Transition93/1
  [G1] -> Rate Transition96/1
  mpc_enable/14(enb_mpc_done) -> Terminator23/1
  [pu_conv_valid] -> uz_vsd_6ph_30deg/7(pu_conv_valid)
  Rate Transition/1 -> Gain/1
  Demux4/1 -> Mux/1  "id"
  Demux4/2 -> Mux/2  "iq"
  6ph_PMSM_30deg_VSD1/3(y3) -> Mux/3  "ix"
  6ph_PMSM_30deg_VSD1/4(y4) -> Mux/4  "iy"
  Rate Transition5/1 -> 6ph_PMSM_30deg_VSD1/7(k6)
  Rate Transition8/1 -> 6ph_PMSM_30deg_VSD1/8(c6)
  Rate Transition131/1 -> Mux5/3
  Rate Transition132/1 -> Alpha-Beta-Zero to dq1/2
  Mux/1 -> Scope/1
  uz_debug_switch_measurements/1(out0) -> [i_a1]
  uz_debug_switch_measurements/2(out1) -> [i_b1]
  uz_debug_switch_measurements/7(out6) -> [v_dc]
  uz_debug_switch_measurements/6(out5) -> [i_c2]
  uz_debug_switch_measurements/5(out4) -> [i_b2]
  uz_debug_switch_measurements/4(out3) -> [i_a2]
  uz_debug_switch_measurements/3(out2) -> [i_c1]
  [i_a1] -> uz_pu_conversion/1(in0)
  [i_b1] -> uz_pu_conversion/2(in1)
  [i_c1] -> uz_pu_conversion/3(in2)
  [i_a2] -> uz_pu_conversion/4(in3)
  [i_b2] -> uz_pu_conversion/5(in4)
  [i_c2] -> uz_pu_conversion/6(in5)
  [v_dc] -> uz_pu_conversion/7(in6)
  uz_debug_switch_measurements/10(debug_ip_done) -> [debug_ip_done]
  [debug_ip_done] -> uz_pu_conversion/15(adc_valid_trigger)
  Rate Transition134/1 -> uz_current_limit/1(ia1_SI)
  Rate Transition133/1 -> uz_current_limit/2(ib1_SI)
  Rate Transition137/1 -> uz_current_limit/3(ic1_SI)
  Rate Transition135/1 -> uz_current_limit/4(ia2_SI)
  Rate Transition136/1 -> uz_current_limit/5(ib2_SI)
  Rate Transition138/1 -> uz_current_limit/6(ic2_SI)
  uz_current_limit/3(done) -> Terminator26/1
  Demux1/2 -> Data Type Conversion72/1
  Demux1/5 -> Data Type Conversion75/1
  Demux1/3 -> Data Type Conversion73/1
  Demux1/1 -> Data Type Conversion71/1
  [i_ph] -> Demux1/1
  Demux1/6 -> Data Type Conversion76/1
  Demux1/4 -> Data Type Conversion74/1
  Data Type Conversion71/1 -> Rate Transition134/1
  Data Type Conversion72/1 -> Rate Transition133/1
  Data Type Conversion73/1 -> Rate Transition137/1
  Data Type Conversion74/1 -> Rate Transition135/1
  Data Type Conversion75/1 -> Rate Transition136/1
  Data Type Conversion76/1 -> Rate Transition138/1
  Rate Transition139/1 -> uz_current_limit/7(i_max_ampere_AXI)
  Data Type Conversion77/1 -> Rate Transition139/1
  Constant16/1 -> Data Type Conversion77/1
  uz_current_limit/1(current_limit_violated) -> [current_limit_violated]
  uz_current_limit/2(current_limit_violated_AXI) -> Terminator28/1
  [current_limit_violated] -> Terminator27/1
  prediction/2(iq_pred_pu) -> [iq_pred_pu]
  Constant23/1 -> Gain1/1
  Constant27/1 -> Data Type Conversion58/1
  Rate Transition140/1 -> mpc_enable/14(overcurrent_disable)
  [current_limit_violated] -> Rate Transition140/1
  Constant36/1 -> [MPC_enb]
  mpc_enable/13(mpc_enb) -> [MPC_enb_out]
  Constant37/1 -> [Inverter_en]
  [MPC_enb_out] -> AND/2
  [Inverter_en] -> AND/1
  Data Type Conversion78/1 -> Transport Delay/1
  Transport Delay/1 -> Data Type Conversion79/1
  Data Type Conversion79/1 -> inverter_machine/2(inverter_en)
  AND/1 -> Data Type Conversion78/1
  Rate Transition141/1 -> uz_current_limit/8(reset_violation_AXI)
  [MPC_enb] -> Rate Transition141/1

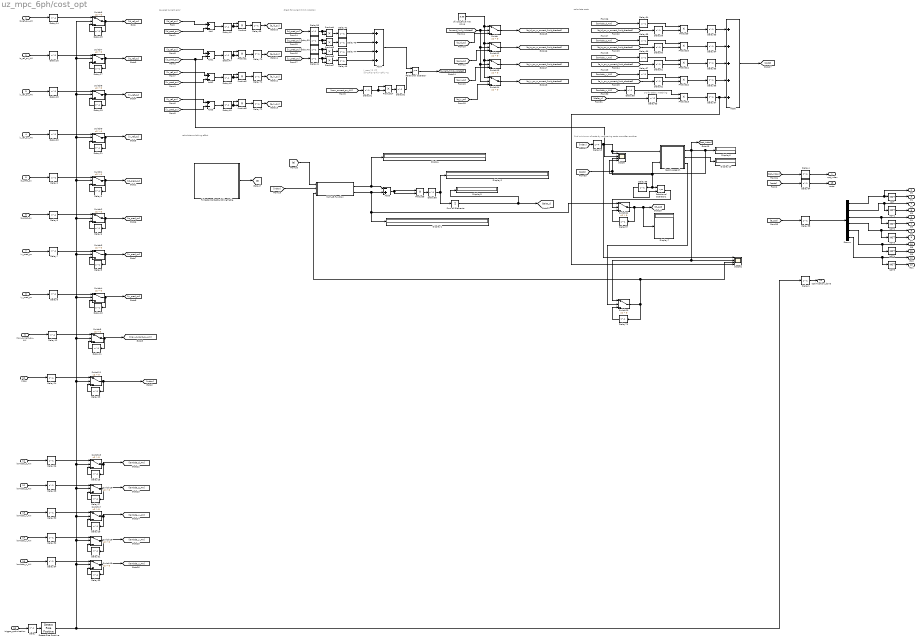
== system uz_mpc_6ph/cost_opt ==
  note: z-2 for delay matching
  note: i_max^2 <= id^2+iq^2+ix^2+iy^2
  note: find minimum of costs by comparing costs one after another
  note: calculate costs
  note: calculate switching effort
  note: check for current limit violation
  note: squared current error
  id_ref_pu_AXI : Inport
  iq_ref_pu_AXI : Inport  Port=2
  ix_ref_pu_AXI : Inport  Port=3
  iy_ref_pu_AXI : Inport  Port=4
  id_pred_pu : Inport  Port=5
  iq_pred_pu : Inport  Port=6
  ix_pred_pu : Inport  Port=7
  iy_pred_pu : Inport  Port=8
  max_current_pu_AXI : Inport  Port=9
  index : Inport  Port=10
  lambda_d_AXI : Inport  Port=11
  lambda_q_AXI : Inport  Port=12
  lambda_x_AXI : Inport  Port=13
  lambda_y_AXI : Inport  Port=14
  lambda_u_AXI : Inport  Port=15
  trigger_optimization : Inport  Port=16
  Add{,1..3} (4 alike) : Sum  Inputs=+-
  Add4 : Sum  Inputs=++++  AccumDataTypeStr=fixdt_type_squared_current_error
  Add5 : Sum  Inputs=-+
  Add6 : Sum  Inputs=+++++  AccumDataTypeStr=fixdt_type_delta_u_costs
  Delay{,1..12,14..21,25..34,36,38..49,51..62,64..72,94} (66 alike) : Delay  DelayLength=1
  Delay13 : Delay  DelayLength=4
  Delay23 : Delay  DelayLength=1  InitialCondition=1
  Delay24 : Delay  DelayLength=1  InitialCondition=1
  Delay35 : Delay  DelayLength=1  InitialCondition=4.99
  Delay37 : Delay  DelayLength=1  InitialCondition=0
  Delay63 : Delay
  Delay73 : Delay  DelayLength=1  InitialCondition=1
  Demux : Demux  Outputs=6
  Detect Rise Positive : simulink/Logic and Bit Operations/Detect Rise Positive  vinit=0  OutDataTypeStr=boolean
  Display{,1..3,6..7,10} (7 alike) : Display
  FiniteControlSetSwitchingTable : MATLAB Function  TreatAsAtomicUnit=on
  MATLAB Function : MATLAB Function  TreatAsAtomicUnit=on
  NOT{,1..5} (6 alike) : Logic  Operator=NOT  IconShape=distinctive  AllPortsSameDT=off  OutDataTypeStr=boolean
  Product{,1..7,9..12,14} (13 alike) : Product  OutDataTypeStr=fixdt_type_squared_current_error
  Product13 : Product  OutDataTypeStr=fixdt_type_delta_u_costs
  Product8 : Product  OutDataTypeStr=uint16
  Relational Operator : RelationalOperator  OutDataTypeStr=boolean  RndMeth=Simplest  InputSameDT=off
  Relational Operator1 : RelationalOperator  Operator=<=  OutDataTypeStr=boolean  RndMeth=Simplest  InputSameDT=off
  Scope : Scope  NumInputPorts=4
  Scope1 : Scope  NumInputPorts=4
  Sum of Elements : Sum  Inputs=+  AccumDataTypeStr=uint16
  Switch{,1..9,11..21} (21 alike) : Switch  Criteria=u2 > Threshold  SaturateOnIntegerOverflow=off  InputSameDT=off
  iterativesearch : MATLAB Function  TreatAsAtomicUnit=on
  sfix18_En15 max value : Constant  Value=3.99  OutDataTypeStr=fixdt(1,18,15)  SampleTime=-1
  opt_index : Outport  VectorParamsAs1DForOutWhenUnconnected=off
  G0 : Outport  Port=2  VectorParamsAs1DForOutWhenUnconnected=off
  G1 : Outport  Port=3  VectorParamsAs1DForOutWhenUnconnected=off
  G2 : Outport  Port=4  VectorParamsAs1DForOutWhenUnconnected=off
  G3 : Outport  Port=5  VectorParamsAs1DForOutWhenUnconnected=off
  G4 : Outport  Port=6  VectorParamsAs1DForOutWhenUnconnected=off
  G5 : Outport  Port=7  VectorParamsAs1DForOutWhenUnconnected=off
  G6 : Outport  Port=8  VectorParamsAs1DForOutWhenUnconnected=off
  G7 : Outport  Port=9  VectorParamsAs1DForOutWhenUnconnected=off
  G8 : Outport  Port=10  VectorParamsAs1DForOutWhenUnconnected=off
  G9 : Outport  Port=11  VectorParamsAs1DForOutWhenUnconnected=off
  G10 : Outport  Port=12  VectorParamsAs1DForOutWhenUnconnected=off
  G11 : Outport  Port=13  VectorParamsAs1DForOutWhenUnconnected=off
  optimization_done : Outport  Port=14  VectorParamsAs1DForOutWhenUnconnected=off
  costs : Outport  Port=15  VectorParamsAs1DForOutWhenUnconnected=off
  wires:
  trigger_optimization/1 -> Delay/1
  Delay/1 -> Detect Rise Positive/1
  Delay1/1 -> optimization_done/1
  Delay4/1 -> opt_index/1
  Switch9/1 -> [iy_ref_pu], Delay21/1
  Delay17/1 -> Switch7/3
  id_ref_pu_AXI/1 -> Delay14/1
  Delay18/1 -> Switch8/1
  Switch8/1 -> [ix_ref_pu], Delay19/1
  Delay21/1 -> Switch9/3
  Switch7/1 -> [iq_ref_pu], Delay17/1
  iy_ref_pu_AXI/1 -> Delay20/1
  iq_ref_pu_AXI/1 -> Delay16/1
  Delay16/1 -> Switch7/1
  Delay19/1 -> Switch8/3
  Delay20/1 -> Switch9/1
  Delay15/1 -> Switch6/3
  Switch6/1 -> [id_ref_pu], Delay15/1
  ix_ref_pu_AXI/1 -> Delay18/1
  Delay14/1 -> Switch6/1
  Switch1/1 -> [id_pred_pu], Delay3/1
  ix_pred_pu/1 -> Delay7/1
  Delay9/1 -> Switch4/1
  Delay2/1 -> Switch1/1
  Delay8/1 -> Switch3/3
  Delay5/1 -> Switch2/1
  iy_pred_pu/1 -> Delay9/1
  iq_pred_pu/1 -> Delay5/1
  Switch3/1 -> Delay8/1, [ix_pred_pu]
  Delay10/1 -> Switch4/3
  Switch2/1 -> [iq_pred_pu], Delay6/1
  Delay7/1 -> Switch3/1
  Switch4/1 -> [iy_pred_pu], Delay10/1
  Delay6/1 -> Switch2/3
  Delay3/1 -> Switch1/3
  id_pred_pu/1 -> Delay2/1
  max_current_pu_AXI/1 -> Delay12/1
  Delay12/1 -> Switch5/1
  Delay11/1 -> Switch5/3
  Switch5/1 -> [max_current_pu_AXI], Delay11/1
  FiniteControlSetSwitchingTable/1(G) -> [G]
  Delay24/1 -> Switch11/1
  index/1 -> Delay24/1
  Delay23/1 -> Switch11/3
  [e_id_pu] -> Switch/3
  [current_limit_violated] -> Switch13/2, Switch14/2, Switch12/2, Switch/2
  [e_iq_pu] -> Switch12/3
  [e_ix_pu] -> Switch13/3
  sfix18_En15 max value/1 -> Switch/1, Switch14/1, Switch13/1, Switch12/1
  [e_iy_pu] -> Switch14/3
  [G] -> MATLAB Function/1(in)
  Delay26/1 -> Switch15/1
  Delay25/1 -> Switch15/3
  Switch15/1 -> [lambda_d_AXI], Delay25/1
  lambda_d_AXI/1 -> Delay26/1
  lambda_q_AXI/1 -> Delay28/1
  Delay28/1 -> Switch16/1
  Switch16/1 -> [lambda_q_AXI], Delay27/1
  Delay27/1 -> Switch16/3
  lambda_y_AXI/1 -> Delay32/1
  Switch18/1 -> [lambda_y_AXI], Delay31/1
  Delay31/1 -> Switch18/3
  Delay32/1 -> Switch18/1
  lambda_x_AXI/1 -> Delay30/1
  Delay30/1 -> Switch17/1
  Switch17/1 -> [lambda_x_AXI], Delay29/1
  Delay29/1 -> Switch17/3
  Delay33/1 -> Switch19/3
  Switch19/1 -> [lambda_u_AXI], Delay33/1
  lambda_u_AXI/1 -> Delay34/1
  Delay34/1 -> Switch19/1
  [opt_index] -> Delay4/1
  Delay38/1 -> Demux/1
  Add4/1 -> Relational Operator/1
  NOT/1 -> G1/1
  Demux/1 -> G0/1, NOT/1
  NOT5/1 -> G11/1
  NOT4/1 -> G9/1
  NOT3/1 -> G7/1
  NOT2/1 -> G5/1
  NOT1/1 -> G3/1
  Demux/2 -> NOT1/1, G2/1
  Demux/3 -> NOT2/1, G4/1
  Demux/4 -> NOT3/1, G6/1
  Demux/5 -> NOT4/1, G8/1
  Demux/6 -> NOT5/1, G10/1
  Product8/1 -> Delay58/1
  Add5/1 -> Product8/1, Product8/2
  MATLAB Function/1(G_next) -> Display/1, Add5/1
  Product9/1 -> Delay53/1
  Product10/1 -> Delay54/1
  Product11/1 -> Delay55/1
  Product12/1 -> Delay56/1
  Product13/1 -> Delay57/1
  Add6/1 -> [costs]
  [lambda_d_AXI] -> Delay64/1
  [lambda_q_AXI] -> Delay65/1
  [lambda_x_AXI] -> Delay66/1
  [lambda_y_AXI] -> Delay67/1
  [lambda_u_AXI] -> Delay68/1
  [delta_u] -> Delay63/1
  [e_id_pu_w_current_limit_checked] -> Delay59/1
  [e_iy_pu_w_current_limit_checked] -> Delay62/1
  [e_ix_pu_w_current_limit_checked] -> Delay61/1
  [e_iq_pu_w_current_limit_checked] -> Delay60/1
  [id_ref_pu] -> Add/1
  [id_pred_pu] -> Add/2
  [iq_pred_pu] -> Scope/2, Add1/2
  [iq_ref_pu] -> Add1/1
  [ix_ref_pu] -> Add2/1
  [ix_pred_pu] -> Add2/2
  [iy_ref_pu] -> Add3/1
  [iy_pred_pu] -> Add3/2
  Add3/1 -> Delay49/1
  Add1/1 -> Delay47/1
  Add2/1 -> Delay48/1
  Add/1 -> Delay46/1
  Product3/1 -> Delay72/1
  Product2/1 -> Delay71/1
  Product1/1 -> Delay70/1
  Product/1 -> Delay69/1
  Product4/1 -> Delay42/1
  Product5/1 -> Delay43/1
  Product6/1 -> Delay44/1
  Product7/1 -> Delay45/1
  [id_pred_pu] -> Delay36/1
  [iq_pred_pu] -> Delay39/1
  [ix_pred_pu] -> Delay40/1
  [iy_pred_pu] -> Delay41/1
  Relational Operator/1 -> [current_limit_violated]
  Switch14/1 -> [e_iy_pu_w_current_limit_checked]
  Switch13/1 -> [e_ix_pu_w_current_limit_checked]
  Switch12/1 -> [e_iq_pu_w_current_limit_checked]
  Switch/1 -> [e_id_pu_w_current_limit_checked]
  [max_current_pu_AXI] -> Delay51/1
  Product14/1 -> Delay52/1
  [costs] -> Delay94/1
  Delay94/1 -> costs/1
  Delay37/1 -> Switch21/3
  Switch21/1 -> Display7/1, [G_opt], Delay37/1
  Detect Rise Positive/1 -> Switch4/2, Switch3/2, Switch2/2, Switch1/2, Switch6/2, Switch7/2, Switch8/2, Switch9/2, Switch5/2, Switch11/2, Switch15/2, Switch16/2, Switch17/2, Switch18/2, Switch19/2, Delay1/1
  [costs] -> Scope/3, Delay35/1, Relational Operator1/1, iterativesearch/2(cost)
  [index] -> Delay13/1  "idx"
  Delay35/1 -> Relational Operator1/2
  Relational Operator1/1 -> Switch21/2
  [G_opt] -> Delay38/1
  Delay36/1 -> Product4/2, Product4/1
  Delay39/1 -> Product5/2, Product5/1
  Delay40/1 -> Product6/2, Product6/1
  Delay41/1 -> Product7/2, Product7/1
  Delay44/1 -> Add4/3
  Delay42/1 -> Add4/1
  Delay45/1 -> Add4/4
  Delay43/1 -> Add4/2
  Delay46/1 -> Product/1, Product/2
  Delay47/1 -> Product1/1, Product1/2
  Delay48/1 -> Product2/1, Product2/2
  Delay49/1 -> Product3/1, Product3/2
  Switch11/1 -> [index], Delay23/1
  Delay51/1 -> Product14/1, Product14/2
  Delay52/1 -> Relational Operator/2
  Delay53/1 -> Add6/1
  Delay54/1 -> Add6/2
  Delay55/1 -> Add6/3
  Delay56/1 -> Add6/4
  Delay57/1 -> Add6/5, Scope1/4  "dU"
  Delay58/1 -> Sum of Elements/1, Display2/1
  Delay59/1 -> Product9/2
  Delay60/1 -> Product10/2
  Delay61/1 -> Product11/2
  Delay62/1 -> Product12/2
  Delay63/1 -> Product13/2
  Delay64/1 -> Product9/1
  Delay65/1 -> Product10/1
  Delay66/1 -> Product11/1
  Delay67/1 -> Product12/1
  Delay68/1 -> Product13/1
  Delay69/1 -> [e_id_pu]
  Delay70/1 -> [e_iq_pu]
  Delay71/1 -> [e_ix_pu]
  Delay72/1 -> [e_iy_pu]
  Sum of Elements/1 -> [delta_u], Display3/1
  Switch20/1 -> Delay73/1, MATLAB Function/3(last_optim_index), Scope1/3  "last_opt_idx"
  MATLAB Function/2(G_prev) -> Display1/1, Switch21/1, Add5/2
  Delay73/1 -> Switch20/3
  iterativesearch/1(opt_idx) -> Scope1/2, Switch20/1, Scope/4, Display6/1, [opt_index]  "opt_idx"
  iterativesearch/3(opt_done) -> Switch20/2
  iterativesearch/2(min_costs) -> Display10/1
  [index] -> MATLAB Function/2(index)
  Delay13/1 -> Scope1/1, iterativesearch/1(index), Scope/1

== system uz_mpc_6ph/counter_f_sw_6ph ==
  note: To avoid unneccessary calcualtions, i divide by 24 on the ARM processor.
  note: Over AXI, 32 Bit are received.
      | However, only one Bit is used.
  note: 1 for one cycle if edge recognized
  note: Since i count now every On and Off Transition for each switch,
      |  i have to divide by 12*2 in order to get the switching frequency
      |  (after dividing by the time).
      | 12 comes from the 12 switches
      | 2 comes from that 1 ON-transition and 1 OFF-transition = 1 switching-cycle
  ss_in_0 : Inport
  ss_in_1 : Inport  Port=2
  ss_in_2 : Inport  Port=3
  ss_in_3 : Inport  Port=4
  ss_in_4 : Inport  Port=5
  ss_in_5 : Inport  Port=6
  ss_in_6 : Inport  Port=7
  ss_in_7 : Inport  Port=8
  ss_in_8 : Inport  Port=9
  ss_in_9 : Inport  Port=10
  ss_in_10 : Inport  Port=11
  ss_in_11 : Inport  Port=12
  bResetAXI : Inport  Port=13
  Count_f_sw : MATLAB Function  TreatAsAtomicUnit=on  VariantControl=(default)
  Detec_edge : Sum  Inputs=+-  OutDataTypeStr=int8  AccumDataTypeStr=int8
  Gain : Gain  Commented=on  Gain=1/(12*2)
  Mux : Mux  Inputs=6
  Mux1 : Mux  Inputs=6
  Mux2 : Mux  Inputs=2
  SS_Old : Delay  DelayLength=1
  Saturation : Saturate  UpperLimit=1  LowerLimit=0  OutMin=[0]  OutMax=[1]  OutDataTypeStr=fixdt(0,1)
  Scope : Scope  NumInputPorts=2
  delay : Delay  DelayLength=1
  reset_old2 : Delay  DelayLength=1
  reset_old_switch1 : Switch  Criteria=u2 ~= 0  SaturateOnIntegerOverflow=off  InputSameDT=off
  switchNumb_AXI : Outport  VectorParamsAs1DForOutWhenUnconnected=off
  switchNumb : Outport  Port=2  VectorParamsAs1DForOutWhenUnconnected=off
  wires:
  ss_in_9/1 -> Mux1/4
  ss_in_6/1 -> Mux1/1
  ss_in_10/1 -> Mux1/5
  ss_in_11/1 -> Mux1/6
  ss_in_8/1 -> Mux1/3
  ss_in_1/1 -> Mux/2
  ss_in_5/1 -> Mux/6
  Saturation/1 -> Count_f_sw/4(bReset), Scope/1
  ss_in_4/1 -> Mux/5
  Mux/1 -> Mux2/1
  ss_in_2/1 -> Mux/3
  ss_in_0/1 -> Mux/1
  Mux2/1 -> SS_Old/1, Count_f_sw/3(ss_v)
  delay/1 -> Count_f_sw/1(switchNumb)
  reset_old2/1 -> Detec_edge/2, reset_old_switch1/3
  Detec_edge/1 -> Saturation/1, reset_old_switch1/2  "1 for one cycle if edge recognized"
  Mux1/1 -> Mux2/2
  reset_old_switch1/1 -> reset_old2/1
  ss_in_7/1 -> Mux1/2
  bResetAXI/1 -> Scope/2, reset_old_switch1/1, Detec_edge/1
  ss_in_3/1 -> Mux/4
  SS_Old/1 -> Count_f_sw/2(ss_v_old)
  Count_f_sw/1(switchNumbOut) -> delay/1, switchNumb_AXI/1, switchNumb/1
